simulink model "ImportWindspeed"  (R2022b)
settings: Solver=VariableStepAuto  StartTime=1  StopTime=10  RelTol=1e-3
settings Model: Creator=jim  LastModifiedBy=jim

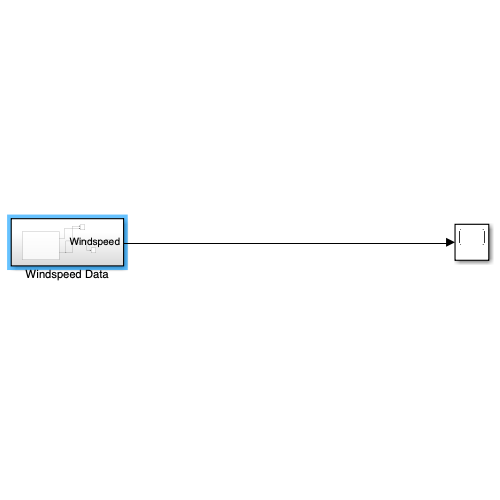
[thumbnail: Simulink's stored preview of the top-level diagram]
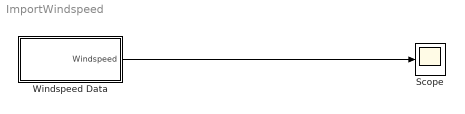
== system ImportWindspeed ==
  Scope : Scope
  Windspeed Data : Subsystem
  wires:
  Windspeed Data/1(Windspeed) -> Scope/1

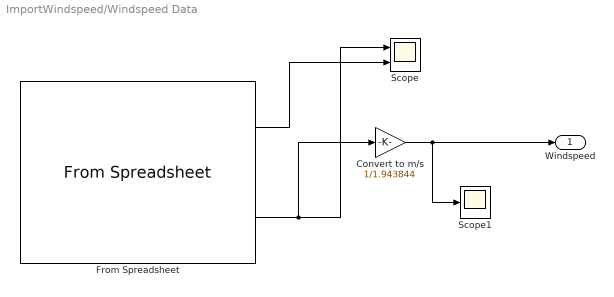
== system ImportWindspeed/Windspeed Data ==
  Convert to m/s : Gain  Gain=1/1.943844
  From Spreadsheet : FromSpreadsheet  FileName=/Users/jim/Dropbox/GitHub Clones/CT549/code/04_Lecture/02 Windspeed/A17_SYN_MACE HEAD_M10_D16.xlsx  SheetName=A17_SYN_MACE HEAD_M10_D16
  Scope : Scope  NumInputPorts=2
  Scope1 : Scope
  Windspeed : Outport
  wires:
  From Spreadsheet/1 -> Scope/2
  From Spreadsheet/2 -> Convert to m/s/1, Scope/1
  Convert to m/s/1 -> Scope1/1, Windspeed/1
